simulink model "Controlabilidad_simu"  (R2021a)
settings: Solver=VariableStepAuto  StartTime=0.0  StopTime=50  FixedStep=1e-6  RelTol=1e-3
values from neighbouring files (symbols this model uses):
  A = [-2 -1; 0 -4]    [Control_Integral.m]    (also in Controlabilidad.m = P.a; Ejemplo_filminas.m = SS.A; Ejercicio_Inestable.m = [100, 0; 160, 200]; Ejercicio_Valvulas.m = double(A))
  B = [1; 0]    [Control_Integral.m]    (also in Controlabilidad.m = P.b; Ejemplo_filminas.m = SS.B; Ejercicio_Inestable.m = [70; 160]; Ejercicio_Valvulas.m = double(B))
  C = [1 1]    [Control_Integral.m]    (also in Controlabilidad.m = P.c; Ejemplo_filminas.m = SS.C; Ejercicio_Inestable.m = [1, 1]; Ejercicio_Valvulas.m = double(C))
  K = [p1-a1 p2-a2] * Wrm * inv(Wr)    [Controlabilidad.m]    (also in Ejemplo_filminas.m; Ejercicio_Inestable.m = [p1 - a1, p2 - a2] * Wrm * inv(Wr); Ejercicio_Valvulas.m = Ka(1:order(P)); realimentacion_ee.m = acker(A, B, [-10 -10]))
  kf = -1/(C*inv(A - B*K) * B)    [Controlabilidad.m]    (also in Ejemplo_filminas.m = -1/(Ccl * inv(Acl)*Bcl); Ejercicio_Inestable.m = 1/(-(C - D*K) * inv(A - B*K) * B + D); realimentacion_ee.m = 10)
settings Model: Creator=Santiago  LastModifiedBy=Santiago

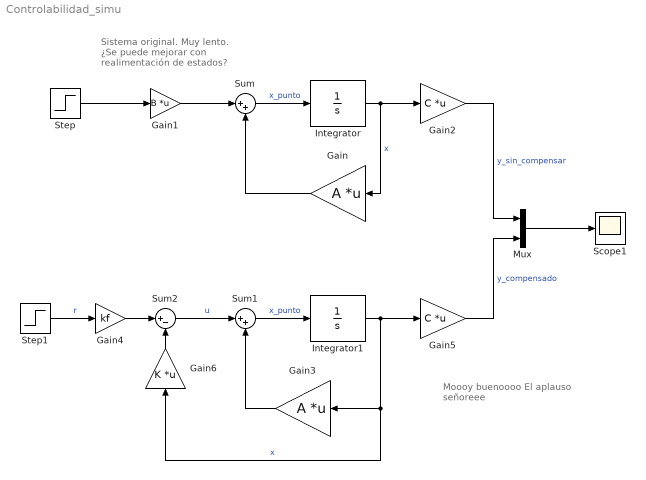
== system Controlabilidad_simu ==
  note: Moooy buenoooo
      | El aplauso señoreee
  note: Sistema original. Muy lento. ¿Se puede mejorar con realimentación de estados?
  Gain : Gain  Gain=A  Multiplication=Matrix(K*u) (u vector)
  Gain1 : Gain  Gain=B  Multiplication=Matrix(K*u)
  Gain2 : Gain  Gain=C  Multiplication=Matrix(K*u) (u vector)
  Gain3 : Gain  Gain=A  Multiplication=Matrix(K*u) (u vector)
  Gain4 : Gain  Gain=kf
  Gain5 : Gain  Gain=C  Multiplication=Matrix(K*u) (u vector)
  Gain6 : Gain  Gain=K  Multiplication=Matrix(K*u) (u vector)
  Integrator : Integrator
  Integrator1 : Integrator
  Mux : Mux  Inputs=2
  Scope1 : Scope
  Step : Step  SampleTime=0
  Step1 : Step  SampleTime=0
  Sum : Sum  Inputs=|++
  Sum1 : Sum  Inputs=|++
  Sum2 : Sum  Inputs=|+-
  wires:
  Gain/1 -> Sum/2
  Gain1/1 -> Sum/1
  Step/1 -> Gain1/1
  Sum/1 -> Integrator/1  "x_punto"
  Integrator/1 -> Gain2/1, Gain/1  "x"
  Gain3/1 -> Sum1/2
  Integrator1/1 -> Gain5/1, Gain6/1, Gain3/1  "x"
  Sum1/1 -> Integrator1/1  "x_punto"
  Gain4/1 -> Sum2/1
  Sum2/1 -> Sum1/1  "u"
  Step1/1 -> Gain4/1  "r"
  Gain6/1 -> Sum2/2
  Mux/1 -> Scope1/1
  Gain2/1 -> Mux/1  "y_sin_compensar"
  Gain5/1 -> Mux/2  "y_compensado"
